simulink model "etsim"  (R2024b)
settings: Solver=VariableStepAuto  StartTime=0.0  StopTime=10.0  RelTol=1e-3
values from neighbouring files (symbols this model uses):
  C_filter = T/(Tc + T)    (= 0.0215179442657)    [BalRob_Params.m]
  K_ET_LQR = K_Nom_LQR_Br    [ET_LQR_Tracking_Setup.m]    (also in et.m)
  lambda_eta_ET = 1.5    [ET_LQR_Tracking_Setup.m]    (also in et.m)
  minSteps_ET = max(1, round(Tmin_ET/Ts))    [ET_LQR_Tracking_Setup.m]    (also in et.m)
  mode_ET = 2    [ET_LQR_Tracking_Setup.m]    (also in et.m)
  P_ET = 0.5*(P_ET + P_ET.')    [ET_LQR_Tracking_Setup.m]    (also in et.m)
  sigma_ET = 0.10    (= 0.1)    [ET_LQR_Tracking_Setup.m]    (also in et.m)
  T = 1e-02    (= 0.01)    [BalRob_Params.m]
  Ts = 1e-2    (= 0.01)    [BalRob_Params.m]
  uMax_ET = drv.Vbus    [ET_LQR_Tracking_Setup.m]    (also in et.m)
undefined symbols (not defined in the file or in its folder): drv, dspblkCoreblockFVToolHelper, gbox, gcbh, sens
settings Model: Creator=marja  LastModifiedBy=marja

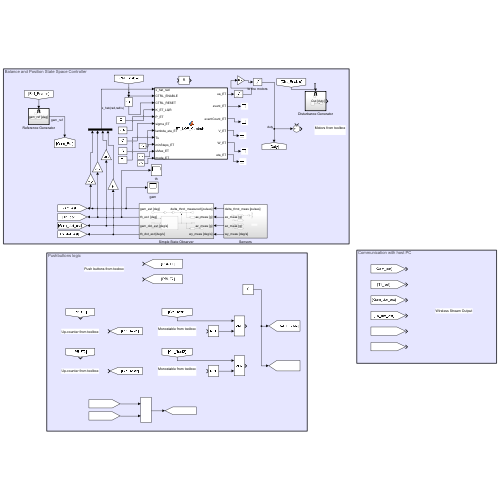
[thumbnail: Simulink's stored preview of the top-level diagram]
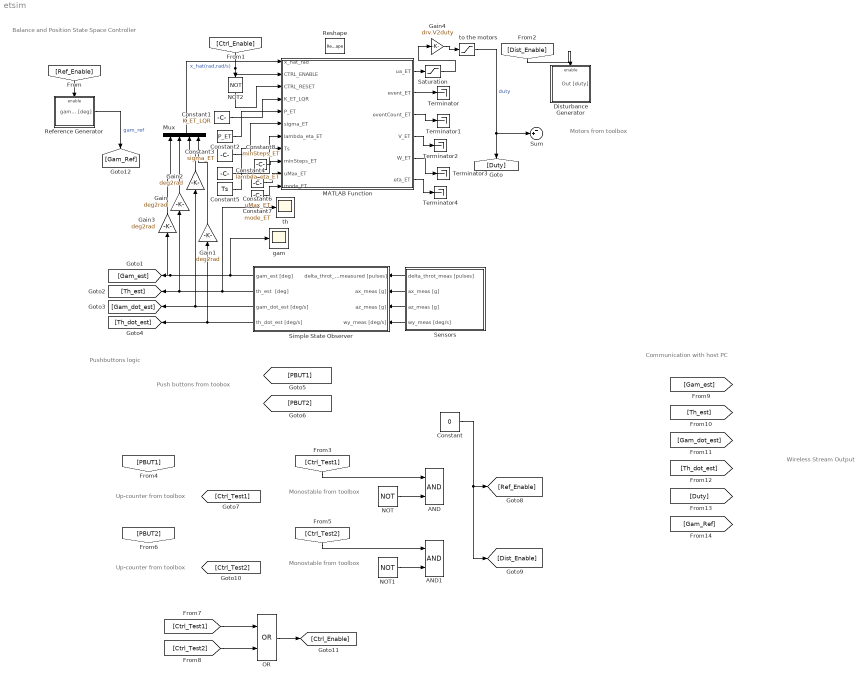
== system etsim ==
  note: Pushbuttons logic
  note: Balance and Position State Space Controller
  note: Up-counter from toolbox
  note: Monostable from toolbox
  note: Push buttons from toobox
  note: Up-counter from toolbox
  note: Wireless Stream Output
  note: Monostable from toolbox
  note: Motors from toolbox
  note: Communication with host PC
  AND : Logic  AllPortsSameDT=off  OutDataTypeStr=boolean
  AND1 : Logic  AllPortsSameDT=off  OutDataTypeStr=boolean
  Constant : Constant  Value=0  SampleTime=0.01
  Constant1 : Constant  Value=K_ET_LQR  SampleTime=Ts
  Constant2 : Constant  Value=P_ET  SampleTime=Ts
  Constant3 : Constant  Value=sigma_ET  SampleTime=Ts
  Constant4 : Constant  Value=lambda_eta_ET  SampleTime=Ts
  Constant5 : Constant  Value=Ts  SampleTime=Ts
  Constant6 : Constant  Value=uMax_ET  SampleTime=Ts
  Constant7 : Constant  Value=mode_ET  SampleTime=Ts
  Constant8 : Constant  Value=minSteps_ET  SampleTime=Ts
  Disturbance Generator : Subsystem
  Gain{,1..3} (4 alike) : Gain  Gain=deg2rad
  Gain4 : Gain  Gain=drv.V2duty
  MATLAB Function : MATLAB Function  TreatAsAtomicUnit=on
  Mux : Mux
  NOT : Logic  Operator=NOT  AllPortsSameDT=off  OutDataTypeStr=boolean
  NOT1 : Logic  Operator=NOT  AllPortsSameDT=off  OutDataTypeStr=boolean
  NOT2 : Logic  Operator=NOT  AllPortsSameDT=off  OutDataTypeStr=boolean
  OR : Logic  Operator=OR  AllPortsSameDT=off  OutDataTypeStr=boolean
  Reference Generator : Subsystem
  Reshape : Reshape  OutputDimensionality=Customize  OutputDimensions=[4,1]
  Saturation : Saturate  UpperLimit=+drv.Vbus  LowerLimit=-drv.Vbus
  Sensors : Subsystem
  Simple State Observer : Subsystem
  Sum : Sum  Inputs=-+|
  Terminator{,1..4} (5 alike) : Terminator
  gam : Scope
  th : Scope
  to the motors : Saturate  UpperLimit=drv.dutymax  LowerLimit=-drv.dutymax
  wires:
  Simple State Observer/3(gam_dot_est [deg/s]) -> [Gam_dot_est], Gain2/1
  Reference Generator/1(gam_ref [deg]) -> [Gam_Ref]  "gam_ref"
  OR/1 -> [Ctrl_Enable]
  Simple State Observer/2(th_est  [deg]) -> th/1, Gain/1, [Th_est]
  Sensors/4(wy_meas [deg/s]) -> Simple State Observer/4(wy_meas [deg/s])
  Sensors/1(delta_throt_meas [pulses]) -> Simple State Observer/1(delta_throt_measured [pulses])
  [Ctrl_Test2] -> OR/2
  [Dist_Enable] -> Disturbance Generator/Enable
  [Ref_Enable] -> Reference Generator/Enable
  to the motors/1 -> Sum/2, [Duty]  "duty"
  Simple State Observer/1(gam_est [deg]) -> gam/1, Gain3/1, [Gam_est]
  NOT1/1 -> AND1/2
  Constant/1 -> [Dist_Enable], [Ref_Enable]
  [Ctrl_Test1] -> OR/1
  NOT/1 -> AND/2
  Simple State Observer/4(th_dot_est [deg/s]) -> [Th_dot_est], Gain1/1
  Sensors/2(ax_meas [g]) -> Simple State Observer/2(ax_meas [g])
  [Ctrl_Test1] -> AND/1
  Sensors/3(az_meas [g]) -> Simple State Observer/3(az_meas [g])
  [Ctrl_Test2] -> AND1/1
  [Ctrl_Enable] -> NOT2/1, MATLAB Function/2(CTRL_ENABLE)
  Gain3/1 -> Mux/1
  Gain/1 -> Mux/2
  Gain2/1 -> Mux/3
  Gain1/1 -> Mux/4
  Mux/1 -> MATLAB Function/1(x_hat_rad)  "x_hat(rad,rad/s)"
  NOT2/1 -> MATLAB Function/3(CTRL_RESET)
  Constant1/1 -> MATLAB Function/4(K_ET_LQR)
  Constant2/1 -> MATLAB Function/5(P_ET)
  Constant3/1 -> MATLAB Function/6(sigma_ET)
  Constant4/1 -> MATLAB Function/7(lambda_eta_ET)
  Constant5/1 -> MATLAB Function/8(Ts)
  Constant6/1 -> MATLAB Function/10(uMax_ET)
  Constant7/1 -> MATLAB Function/11(mode_ET)
  Constant8/1 -> MATLAB Function/9(minSteps_ET)
  MATLAB Function/1(ua_ET) -> Saturation/1
  Saturation/1 -> Gain4/1
  Gain4/1 -> to the motors/1
  MATLAB Function/2(event_ET) -> Terminator/1
  MATLAB Function/3(eventCount_ET) -> Terminator1/1
  MATLAB Function/4(V_ET) -> Terminator2/1
  MATLAB Function/5(W_ET) -> Terminator3/1
  MATLAB Function/6(eta_ET) -> Terminator4/1

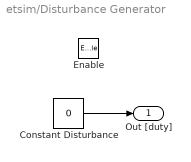
== system etsim/Disturbance Generator ==
  Enable : EnablePort
  Constant Disturbance : Constant  Value=0
  Out [duty] : Outport  OutputWhenDisabled=reset  InitialOutput=0
  wires:
  Constant Disturbance/1 -> Out [duty]/1

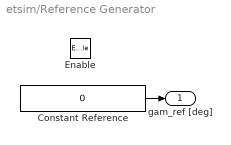
== system etsim/Reference Generator ==
  Enable : EnablePort
  Constant Reference : Constant  Value=0
  gam_ref [deg] : Outport  OutputWhenDisabled=reset  InitialOutput=0
  wires:
  Constant Reference/1 -> gam_ref [deg]/1

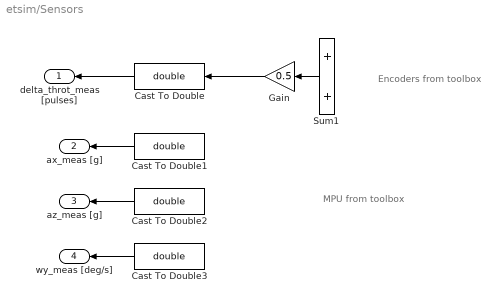
== system etsim/Sensors ==
  note: Encoders from toolbox
  note: MPU from toolbox
  Cast To Double{,1..3} (4 alike) : DataTypeConversion  OutDataTypeStr=double  SaturateOnIntegerOverflow=off  RndMeth=Floor
  Gain : Gain  Gain=0.5
  Sum1 : Sum
  delta_throt_meas [pulses] : Outport
  ax_meas [g] : Outport  Port=2
  az_meas [g] : Outport  Port=3
  wy_meas [deg/s] : Outport  Port=4
  wires:
  Sum1/1 -> Gain/1
  Gain/1 -> Cast To Double/1
  Cast To Double/1 -> delta_throt_meas [pulses]/1
  Cast To Double3/1 -> wy_meas [deg/s]/1
  Cast To Double2/1 -> az_meas [g]/1
  Cast To Double1/1 -> ax_meas [g]/1

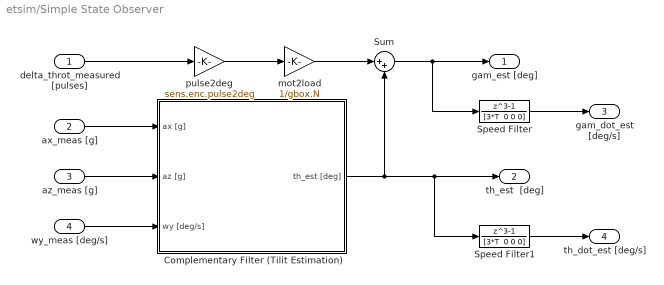
== system etsim/Simple State Observer ==
  delta_throt_measured [pulses] : Inport
  ax_meas [g] : Inport  Port=2
  az_meas [g] : Inport  Port=3
  wy_meas [deg/s] : Inport  Port=4
  Complementary Filter (Tilit Estimation) : Subsystem
  Speed Filter : DiscreteTransferFcn  LoadFcn=dspblkCoreblockFVToolHelper(gcbh,'load');  Numerator=[1 0 0 -1]  Denominator="[3*T  0 0 0]"
      settings: CopyFcn=dspblkCoreblockFVToolHelper(gcbh,'copy');  DeleteFcn=dspblkCoreblockFVToolHelper(gcbh,'close');  ModelCloseFcn=dspblkCoreblockFVToolHelper(gcbh,'close');  PreSaveFcn=dspblkCoreblockFVToolHelper(gcbh,'presave');  PostSaveFcn=dspblkCoreblockFVToolHelper(gcbh,'postsave');  CloseFcn=dspblkCoreblockFVToolHelper(gcbh,'close');
  Speed Filter1 : DiscreteTransferFcn  LoadFcn=dspblkCoreblockFVToolHelper(gcbh,'load');  Numerator=[1 0 0 -1]  Denominator="[3*T  0 0 0]"
      settings: CopyFcn=dspblkCoreblockFVToolHelper(gcbh,'copy');  DeleteFcn=dspblkCoreblockFVToolHelper(gcbh,'close');  ModelCloseFcn=dspblkCoreblockFVToolHelper(gcbh,'close');  PreSaveFcn=dspblkCoreblockFVToolHelper(gcbh,'presave');  PostSaveFcn=dspblkCoreblockFVToolHelper(gcbh,'postsave');  CloseFcn=dspblkCoreblockFVToolHelper(gcbh,'close');
  Sum : Sum  Inputs=|++
  mot2load : Gain  Gain=1/gbox.N
  pulse2deg : Gain  Gain=sens.enc.pulse2deg
  gam_est [deg] : Outport
  th_est  [deg] : Outport  Port=2
  gam_dot_est [deg/s] : Outport  Port=3
  th_dot_est [deg/s] : Outport  Port=4
  wires:
  mot2load/1 -> Sum/1
  Complementary Filter (Tilit Estimation)/1(th_est [deg]) -> th_est  [deg]/1, Speed Filter1/1, Sum/2
  Speed Filter1/1 -> th_dot_est [deg/s]/1
  delta_throt_measured [pulses]/1 -> pulse2deg/1
  Speed Filter/1 -> gam_dot_est [deg/s]/1
  pulse2deg/1 -> mot2load/1
  Sum/1 -> gam_est [deg]/1, Speed Filter/1
  ax_meas [g]/1 -> Complementary Filter (Tilit Estimation)/1(ax [g])
  az_meas [g]/1 -> Complementary Filter (Tilit Estimation)/2(az [g])
  wy_meas [deg/s]/1 -> Complementary Filter (Tilit Estimation)/3(wy [deg/s])

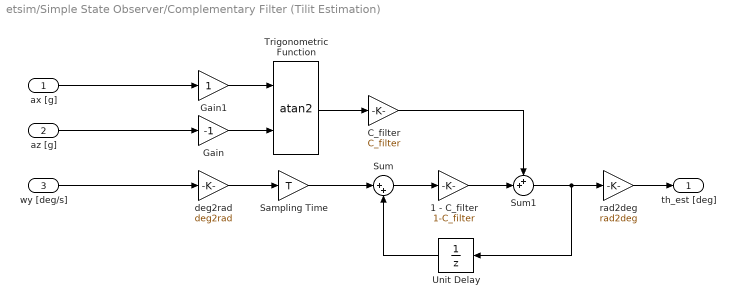
== system etsim/Simple State Observer/Complementary Filter (Tilit Estimation) ==
  ax [g] : Inport
  az [g] : Inport  Port=2
  wy [deg/s] : Inport  Port=3
  1 - C_filter : Gain  Gain=1-C_filter
  C_filter : Gain  Gain=C_filter
  Gain : Gain  Gain=-1
  Gain1 : Gain
  Sampling Time : Gain  Gain=T
  Sum : Sum  Inputs=|++
  Sum1 : Sum  Inputs=++|
  Trigonometric Function : Trigonometry  Operator=atan2
  Unit Delay : UnitDelay  SampleTime=T  HasFrameUpgradeWarning=on
  deg2rad : Gain  Gain=deg2rad
  rad2deg : Gain  Gain=rad2deg
  th_est [deg] : Outport
  wires:
  Trigonometric Function/1 -> C_filter/1
  Gain/1 -> Trigonometric Function/2
  rad2deg/1 -> th_est [deg]/1
  deg2rad/1 -> Sampling Time/1
  Sum/1 -> 1 - C_filter/1
  Gain1/1 -> Trigonometric Function/1
  Sum1/1 -> Unit Delay/1, rad2deg/1
  Sampling Time/1 -> Sum/1
  1 - C_filter/1 -> Sum1/2
  Unit Delay/1 -> Sum/2
  C_filter/1 -> Sum1/1
  ax [g]/1 -> Gain1/1
  az [g]/1 -> Gain/1
  wy [deg/s]/1 -> deg2rad/1

== matlab function etsim/MATLAB Function ==
  data: x_hat_rad input; ua_ET output; CTRL_ENABLE input; CTRL_RESET input; K_ET_LQR input; P_ET input; sigma_ET input; lambda_eta_ET input; Ts input; minSteps_ET input; uMax_ET input; mode_ET input; event_ET output; eventCount_ET output; V_ET output; W_ET output; eta_ET output
function [ua_ET,event_ET,eventCount_ET,V_ET,W_ET,eta_ET] = ET_LQR_Controller( ...
    x_hat_rad, CTRL_ENABLE, CTRL_RESET, K_ET_LQR, P_ET, ...
    sigma_ET, lambda_eta_ET, Ts, minSteps_ET, uMax_ET, mode_ET)
%#codegen
% Practical event-triggered LQR for balancing robot near upright.
%
% Inputs:
%   x_hat_rad     = [gam_est; th_est; dot_gam_est; dot_th_est]
%                   units: [rad; rad; rad/s; rad/s]
%   CTRL_ENABLE   = 1 when controller is enabled
%   CTRL_RESET    = 1 to reset stored event-trigger states
%   K_ET_LQR      = nominal LQR gain, normally K_Nom_LQR_Br
%   P_ET          = Lyapunov matrix from ET_LQR_Setup.m
%   sigma_ET      = event threshold parameter
%   lambda_eta_ET = eta decay rate for V-A
%   Ts            = sample time
%   minSteps_ET   = minimum number of samples between events
%   uMax_ET       = voltage saturation, normally drv.Vbus
%   mode_ET       = 1: V-A, 2: V-C
%
% Outputs:
%   ua_ET         = held motor voltage command [V]
%   event_ET      = 1 only at event/update samples
%   eventCount_ET = total number of control updates/events
%   V_ET          = Lyapunov value V(x)
%   W_ET          = error measure W(e)
%   eta_ET        = threshold variable eta

persistent x_sample_ET ua_hold_ET eventCounter_ET eta_hold_ET ...
           samplesSinceEvent_ET initialized_ET

if isempty(initialized_ET)
    x_sample_ET = zeros(4,1);
    ua_hold_ET = 0;
    eventCounter_ET = uint32(0);
    eta_hold_ET = 0;
    samplesSinceEvent_ET = int32(0);
    initialized_ET = false;
end

event_ET = false;

%% Reset when disabled or manually reset
if CTRL_RESET || ~CTRL_ENABLE
    x_sample_ET = x_hat_rad;
    ua_hold_ET = 0;
    eventCounter_ET = uint32(0);
    eta_hold_ET = 0;
    samplesSinceEvent_ET = int32(0);
    initialized_ET = false;

    ua_ET = ua_hold_ET;
    eventCount_ET = eventCounter_ET;
    V_ET = 0;
    W_ET = 0;
    eta_ET = eta_hold_ET;
    return;
end

%% First active sample: force one control update
if ~initialized_ET
    x_sample_ET = x_hat_rad;

    ua_hold_ET = -K_ET_LQR*x_sample_ET;

    if ua_hold_ET > uMax_ET
        ua_hold_ET = uMax_ET;
    elseif ua_hold_ET < -uMax_ET
        ua_hold_ET = -uMax_ET;
    end

    eventCounter_ET = uint32(1);
    eta_hold_ET = 0;
    samplesSinceEvent_ET = int32(0);
    initialized_ET = true;
    event_ET = true;

    ua_ET = ua_hold_ET;
    eventCount_ET = eventCounter_ET;
    V_ET = x_hat_rad.'*P_ET*x_hat_rad;
    W_ET = 0;
    eta_ET = eta_hold_ET;
    return;
end

%% Sampling-induced state error
% e = last transmitted/sample state - current estimated state
e_ET = x_sample_ET - x_hat_rad;

%% Lyapunov and error measures
V_ET = x_hat_rad.'*P_ET*x_hat_rad;

sigma2_ET = sigma_ET*sigma_ET;
if sigma2_ET < 1e-8
    sigma2_ET = 1e-8;
end

W_ET = (e_ET.'*P_ET*e_ET)/sigma2_ET;

%% Eta dynamics for V-A
% eta_dot = -lambda_eta_ET * eta
eta_hold_ET = eta_hold_ET - Ts*lambda_eta_ET*eta_hold_ET;

if eta_hold_ET < 0
    eta_hold_ET = 0;
end

samplesSinceEvent_ET = samplesSinceEvent_ET + 1;

%% Minimum inter-event time
allowEvent_ET = samplesSinceEvent_ET >= int32(minSteps_ET);

trigger_ET = false;

if allowEvent_ET
    if mode_ET == 1
        % V-A: W(e) >= max(V(x), eta)
        threshold_ET = V_ET;
        if eta_hold_ET > threshold_ET
            threshold_ET = eta_hold_ET;
        end

        trigger_ET = W_ET >= threshold_ET;
    else
        % V-C: W(e) >= V(x)
        trigger_ET = W_ET >= V_ET;
    end
end

%% Event update
if trigger_ET
    W_pre_ET = W_ET;

    x_sample_ET = x_hat_rad;
    ua_hold_ET = -K_ET_LQR*x_sample_ET;

    if ua_hold_ET > uMax_ET
        ua_hold_ET = uMax_ET;
    elseif ua_hold_ET < -uMax_ET
        ua_hold_ET = -uMax_ET;
    end

    eventCounter_ET = eventCounter_ET + uint32(1);
    samplesSinceEvent_ET = int32(0);
    event_ET = true;

    if mode_ET == 1
        % V-A reset: eta^+ = W(e_pre)
        eta_hold_ET = W_pre_ET;
    end
end

%% Outputs
ua_ET = ua_hold_ET;
eventCount_ET = eventCounter_ET;
eta_ET = eta_hold_ET;
